simulink model "sim_tcyb_2024_pos_ctrl"  (R2020a)
settings: Solver=ode4  StartTime=0.0  StopTime=30.0  FixedStep=0.01  RelTol=1e-3
values from neighbouring files (symbols this model uses):
  alfa_theta = 20    [init_tcyb_2024_pos_ctrl.m]
  alfa_theta_obs = 100    [init_tcyb_2024_pos_ctrl.m]
  c1_diff_sigma_bar_v = diag([25; 30; 20])    [init_tcyb_2024_pos_ctrl.m]
  c1v = diag([5.8; 6.5; 6.5])    [init_tcyb_2024_pos_ctrl.m]
  c2_diff_sigma_bar_v = diag([50; 50; 10])    [init_tcyb_2024_pos_ctrl.m]
  c2v = diag([5.8; 6.5; 6.5])    [init_tcyb_2024_pos_ctrl.m]
  c3_diff_sigma_bar_v = diag([15; 15; 10])    [init_tcyb_2024_pos_ctrl.m]
  c3v = diag([4.8; 6.4; 6.0])    [init_tcyb_2024_pos_ctrl.m]
  c_psi_p = [0.05; 0.05; 0.05]    [init_tcyb_2024_pos_ctrl.m]
  delta_p_i_0 = zeros(3, NF)    [init_tcyb_2024_pos_ctrl.m]
  delta_v_i_0 = zeros(3, NF)    [init_tcyb_2024_pos_ctrl.m]
  dp_aa_t = 0.2 * ones(3, 5) + ( 1.0 - 0.2 ) * rand(3, 5)    [init_tcyb_2024_pos_ctrl.m]
  dp_ff_t = [ 0.4 * ones(1, 5) + ( 1.0 - 0.4 ) * rand(1, 5);                      0.4 * ones(1, 5) + ( 1.0 - 0.4 ) * rand(1, 5);                      0.2 * ones(1, 5) + ( 0.6 - 0.2 ) * rand(1, 5) ]    [init_tcyb_2024_pos_ctrl.m]
  dp_phi_t = ( - pi / 2 ) * ones(3, 5) + ( pi / 2 - ( - pi / 2 ) ) * rand(3, 5)    [init_tcyb_2024_pos_ctrl.m]
  etai_0 = zeros(3,5)    [init_tcyb_2024_pos_ctrl.m]
  kai_1_t = 0.02    [init_tcyb_2024_pos_ctrl.m]
  kai_3_t = 0.1    [init_tcyb_2024_pos_ctrl.m]
  ksii_0 = zeros(3,5)    [init_tcyb_2024_pos_ctrl.m]
  l1v = diag([20; 20; 20])    [init_tcyb_2024_pos_ctrl.m]
  l2v = diag([30; 30; 30])    [init_tcyb_2024_pos_ctrl.m]
  Lamd_diff_sigma_bar_v = 0.5    [init_tcyb_2024_pos_ctrl.m]
  mass_i = zeros(1,NF)    [init_tcyb_2024_pos_ctrl.m]
  Mii = diag([1;0;0;0;1])    [init_tcyb_2024_pos_ctrl.m]
  pos0 = zeros(3, 1)    [init_tcyb_2024_pos_ctrl.m]
  PZ0 = P0(3)    [init_tcyb_2024_pos_ctrl.m]
  PZ1 = 10    [init_tcyb_2024_pos_ctrl.m]
  Qci_init = repmat([1;0;0;0],1,NF)    [init_tcyb_2024_pos_ctrl.m]
  R0 = 4    [init_tcyb_2024_pos_ctrl.m]
  R1 = 8    [init_tcyb_2024_pos_ctrl.m]
  rho_p = [0.1; 0.1; 0.1]    [init_tcyb_2024_pos_ctrl.m]
  Rx2 = 10    [init_tcyb_2024_pos_ctrl.m]
  Ry2 = 6    [init_tcyb_2024_pos_ctrl.m]
  Rz2 = 4    [init_tcyb_2024_pos_ctrl.m]
  T0 = 0    [init_tcyb_2024_pos_ctrl.m]
  T1 = tseq1    (= 10)    [init_tcyb_2024_pos_ctrl.m]
  T12 = tseq1 + tseq12    (= 20)    [init_tcyb_2024_pos_ctrl.m]
  T2 = tseq1 + tseq12 + tseq2    (= 30)    [init_tcyb_2024_pos_ctrl.m]
  tau_p = 5    [init_tcyb_2024_pos_ctrl.m]
  theta0 = ( 2 / 5 ) * pi    (= 1.25663706144)    [init_tcyb_2024_pos_ctrl.m]
  vel0 = zeros(3, 1)    [init_tcyb_2024_pos_ctrl.m]
  Wij = [0,0,1,0,0;              0,0,1,1,0;              1,0,0,0,1;              0,1,1,0,0;              0,0,1,0,0]    [init_tcyb_2024_pos_ctrl.m]
  X1 = 8    [init_tcyb_2024_pos_ctrl.m]
  X2 = 2    [init_tcyb_2024_pos_ctrl.m]
  X3 = 3    [init_tcyb_2024_pos_ctrl.m]
  Y1 = 10    [init_tcyb_2024_pos_ctrl.m]
  Y2 = 2    [init_tcyb_2024_pos_ctrl.m]
  Y3 = 4    [init_tcyb_2024_pos_ctrl.m]
  Z1 = 4    [init_tcyb_2024_pos_ctrl.m]
  Z2 = -6    [init_tcyb_2024_pos_ctrl.m]
  Z3 = 2    [init_tcyb_2024_pos_ctrl.m]
  zeta_diff_sigma_bar_v = 0.08    [init_tcyb_2024_pos_ctrl.m]
undefined symbols (not defined in the file or in its folder): cal_frac_squ, p_alfav1, p_alfav2, p_gamma1_pos, p_gamma1_vel, p_gamma2_pos, p_gamma2_vel, q_alfav1, q_alfav2, q_gamma1_pos, q_gamma1_vel, q_gamma2_pos, q_gamma2_vel
(part 3 of 4)

== matlab function sim_tcyb_2024_pos_ctrl/cal theta_sigma_bar_v_tilt agent 3 ==
  data: alfa_theta input; sigma_bar_v_tilt_squ_1_3 input; theta_sigma_bar_v_tilt_1_3 output; sigma_bar_v_tilt_squ_2_3 input; sigma_bar_v_tilt_vec input; theta_sigma_bar_v_tilt_2_3 output
function [theta_sigma_bar_v_tilt_1_3, theta_sigma_bar_v_tilt_2_3] = fcn(alfa_theta, sigma_bar_v_tilt_squ_1_3, sigma_bar_v_tilt_squ_2_3, sigma_bar_v_tilt_vec)
%%%% 计算平滑递增函数
iiuav = 3;
theta_sigma_bar_v_tilt_1_3 = sigma_bar_v_tilt_squ_1_3(:) .* ( -1 + 2 ./ ( 1 + exp( -alfa_theta .* sigma_bar_v_tilt_vec(:,iiuav) ) ) );
theta_sigma_bar_v_tilt_2_3 = sigma_bar_v_tilt_squ_2_3(:) .* ( -1 + 2 ./ ( 1 + exp( -alfa_theta .* sigma_bar_v_tilt_vec(:,iiuav) ) ) );

== matlab function sim_tcyb_2024_pos_ctrl/choose ksi_est_err 25 ==
  data: x input; y output
function y = fcn(x)
iiuav = 3;
y = x(:,iiuav);

== matlab function sim_tcyb_2024_pos_ctrl/choose ksi_est_err 26 ==
  data: x input; y output
function y = fcn(x)
iiuav = 3;
y = x(:,iiuav);

== matlab function sim_tcyb_2024_pos_ctrl/trans to column24 ==
  data: x input; y output
function y = fcn(x)
y = x(:);

== matlab function sim_tcyb_2024_pos_ctrl/trans to column25 ==
  data: x input; y output
function y = fcn(x)
y = x(:);

== matlab function sim_tcyb_2024_pos_ctrl/cal abs 27 ==
  data: x input; y output
function y = fcn(x)
y = abs(x(:));

== matlab function sim_tcyb_2024_pos_ctrl/cal abs 28 ==
  data: x input; y output
function y = fcn(x)
y = abs(x(:));

== matlab function sim_tcyb_2024_pos_ctrl/cal theta_sigma_bar_v_tilt agent 4 ==
  data: alfa_theta input; sigma_bar_v_tilt_squ_1_4 input; theta_sigma_bar_v_tilt_1_4 output; sigma_bar_v_tilt_squ_2_4 input; sigma_bar_v_tilt_vec input; theta_sigma_bar_v_tilt_2_4 output
function [theta_sigma_bar_v_tilt_1_4, theta_sigma_bar_v_tilt_2_4] = fcn(alfa_theta, sigma_bar_v_tilt_squ_1_4, sigma_bar_v_tilt_squ_2_4, sigma_bar_v_tilt_vec)
%%%% 计算平滑递增函数
iiuav = 4;
theta_sigma_bar_v_tilt_1_4 = sigma_bar_v_tilt_squ_1_4(:) .* ( -1 + 2 ./ ( 1 + exp( -alfa_theta .* sigma_bar_v_tilt_vec(:,iiuav) ) ) );
theta_sigma_bar_v_tilt_2_4 = sigma_bar_v_tilt_squ_2_4(:) .* ( -1 + 2 ./ ( 1 + exp( -alfa_theta .* sigma_bar_v_tilt_vec(:,iiuav) ) ) );

== matlab function sim_tcyb_2024_pos_ctrl/choose ksi_est_err 27 ==
  data: x input; y output
function y = fcn(x)
iiuav = 4;
y = x(:,iiuav);

== matlab function sim_tcyb_2024_pos_ctrl/choose ksi_est_err 28 ==
  data: x input; y output
function y = fcn(x)
iiuav = 4;
y = x(:,iiuav);

== matlab function sim_tcyb_2024_pos_ctrl/cal lump formation error ==
  data: err_ksi_form_vec input; err_lump_vec output; err_eta_form_vec input
function err_lump_vec = fcn(err_ksi_form_vec, err_eta_form_vec)
%%%% 计算编队跟踪误差
err_lump_vec = zeros(3,5);
for iiuav = 1:5
    err_lump_vec(:,iiuav) = err_ksi_form_vec(:,iiuav) + err_eta_form_vec(:,iiuav);
end

== matlab function sim_tcyb_2024_pos_ctrl/trans to column26 ==
  data: x input; y output
function y = fcn(x)
y = x(:);

== matlab function sim_tcyb_2024_pos_ctrl/trans to column27 ==
  data: x input; y output
function y = fcn(x)
y = x(:);

== matlab function sim_tcyb_2024_pos_ctrl/cal abs 29 ==
  data: x input; y output
function y = fcn(x)
y = abs(x(:));

== matlab function sim_tcyb_2024_pos_ctrl/cal abs 30 ==
  data: x input; y output
function y = fcn(x)
y = abs(x(:));

== matlab function sim_tcyb_2024_pos_ctrl/cal theta_sigma_bar_v_tilt agent 5 ==
  data: alfa_theta input; sigma_bar_v_tilt_squ_1_5 input; theta_sigma_bar_v_tilt_1_5 output; sigma_bar_v_tilt_squ_2_5 input; sigma_bar_v_tilt_vec input; theta_sigma_bar_v_tilt_2_5 output
function [theta_sigma_bar_v_tilt_1_5, theta_sigma_bar_v_tilt_2_5] = fcn(alfa_theta, sigma_bar_v_tilt_squ_1_5, sigma_bar_v_tilt_squ_2_5, sigma_bar_v_tilt_vec)
%%%% 计算平滑递增函数
iiuav = 5;
theta_sigma_bar_v_tilt_1_5 = sigma_bar_v_tilt_squ_1_5(:) .* ( -1 + 2 ./ ( 1 + exp( -alfa_theta .* sigma_bar_v_tilt_vec(:,iiuav) ) ) );
theta_sigma_bar_v_tilt_2_5 = sigma_bar_v_tilt_squ_2_5(:) .* ( -1 + 2 ./ ( 1 + exp( -alfa_theta .* sigma_bar_v_tilt_vec(:,iiuav) ) ) );

== matlab function sim_tcyb_2024_pos_ctrl/choose ksi_est_err 29 ==
  data: x input; y output
function y = fcn(x)
iiuav = 5;
y = x(:,iiuav);

== matlab function sim_tcyb_2024_pos_ctrl/choose ksi_est_err 30 ==
  data: x input; y output
function y = fcn(x)
iiuav = 5;
y = x(:,iiuav);

== matlab function sim_tcyb_2024_pos_ctrl/trans to column28 ==
  data: x input; y output
function y = fcn(x)
y = x(:);

== matlab function sim_tcyb_2024_pos_ctrl/trans to column29 ==
  data: x input; y output
function y = fcn(x)
y = x(:);

== matlab function sim_tcyb_2024_pos_ctrl/combine theta_sigma_bar_v_tilt ==
  data: theta_sigma_bar_v_tilt_1_1 input; theta_sigma_bar_v_tilt_1_2 input; theta_sigma_bar_v_tilt_1_3 input; theta_sigma_bar_v_tilt_1_4 input; theta_sigma_bar_v_tilt_1_5 input; theta_sigma_bar_v_tilt_1_vec output; theta_sigma_bar_v_tilt_2_1 input; theta_sigma_bar_v_tilt_2_vec output; theta_sigma_bar_v_tilt_2_2 input; theta_sigma_bar_v_tilt_2_3 input; theta_sigma_bar_v_tilt_2_4 input; theta_sigma_bar_v_tilt_2_5 input
function [theta_sigma_bar_v_tilt_1_vec, theta_sigma_bar_v_tilt_2_vec]  = fcn(theta_sigma_bar_v_tilt_1_1, theta_sigma_bar_v_tilt_1_2, theta_sigma_bar_v_tilt_1_3, theta_sigma_bar_v_tilt_1_4, theta_sigma_bar_v_tilt_1_5, ...
                                                                                                                                            theta_sigma_bar_v_tilt_2_1, theta_sigma_bar_v_tilt_2_2, theta_sigma_bar_v_tilt_2_3, theta_sigma_bar_v_tilt_2_4, theta_sigma_bar_v_tilt_2_5)
%%%% 合并领导者位置观测器输出结果
theta_sigma_bar_v_tilt_1_vec = [theta_sigma_bar_v_tilt_1_1(:), theta_sigma_bar_v_tilt_1_2(:), theta_sigma_bar_v_tilt_1_3(:), theta_sigma_bar_v_tilt_1_4(:), theta_sigma_bar_v_tilt_1_5(:)];
theta_sigma_bar_v_tilt_2_vec = [theta_sigma_bar_v_tilt_2_1(:), theta_sigma_bar_v_tilt_2_2(:), theta_sigma_bar_v_tilt_2_3(:), theta_sigma_bar_v_tilt_2_4(:), theta_sigma_bar_v_tilt_2_5(:)];

== matlab function sim_tcyb_2024_pos_ctrl/eps_p_hat adaptive law agent 1 ==
  data: rho_p input; d_eps_p_hat_1 output; err_lump_vec input
function d_eps_p_hat_1 = fcn(rho_p, err_lump_vec)
%%%% 计算自适应律
iiuav = 1;
d_eps_p_hat_1 = ( rho_p(:) .* err_lump_vec(:,iiuav) )' * err_lump_vec(:,iiuav);

== matlab function sim_tcyb_2024_pos_ctrl/cal sigma_bar_v_hat agent 1 ==
  data: c1v input; c2v input; theta_sigma_bar_v_tilt_1_vec input; d_sigma_bar_v_hat_1 output; theta_sigma_bar_v_tilt_2_vec input; d_sigma_bar_v_vec input
function d_sigma_bar_v_hat_1 = fcn(c1v, c2v, theta_sigma_bar_v_tilt_1_vec, theta_sigma_bar_v_tilt_2_vec, d_sigma_bar_v_vec)
%%%% 计算扰动观测器中虚拟速度控制量观测值sigma_v_hat的微分方程
iiuav = 1;
d_sigma_bar_v_hat_1 = d_sigma_bar_v_vec(:,iiuav) + ...
                                            c1v * theta_sigma_bar_v_tilt_1_vec(:,iiuav) + ...
                                            c2v * theta_sigma_bar_v_tilt_2_vec(:,iiuav);

== matlab function sim_tcyb_2024_pos_ctrl/cal sigma_bar_v_hat agent 2 ==
  data: c1v input; c2v input; theta_sigma_bar_v_tilt_1_vec input; d_sigma_bar_v_hat_2 output; theta_sigma_bar_v_tilt_2_vec input; d_sigma_bar_v_vec input
function d_sigma_bar_v_hat_2 = fcn(c1v, c2v, theta_sigma_bar_v_tilt_1_vec, theta_sigma_bar_v_tilt_2_vec, d_sigma_bar_v_vec)
%%%% 计算扰动观测器中虚拟速度控制量观测值sigma_v_hat的微分方程
iiuav = 2;
d_sigma_bar_v_hat_2 = d_sigma_bar_v_vec(:,iiuav) + ...
                                            c1v * theta_sigma_bar_v_tilt_1_vec(:,iiuav) + ...
                                            c2v * theta_sigma_bar_v_tilt_2_vec(:,iiuav);

== matlab function sim_tcyb_2024_pos_ctrl/cal sigma_bar_v_hat agent 3 ==
  data: c1v input; c2v input; theta_sigma_bar_v_tilt_1_vec input; d_sigma_bar_v_hat_3 output; theta_sigma_bar_v_tilt_2_vec input; d_sigma_bar_v_vec input
function d_sigma_bar_v_hat_3 = fcn(c1v, c2v, theta_sigma_bar_v_tilt_1_vec, theta_sigma_bar_v_tilt_2_vec, d_sigma_bar_v_vec)
%%%% 计算扰动观测器中虚拟速度控制量观测值sigma_v_hat的微分方程
iiuav = 3;
d_sigma_bar_v_hat_3 = d_sigma_bar_v_vec(:,iiuav) + ...
                                            c1v * theta_sigma_bar_v_tilt_1_vec(:,iiuav) + ...
                                            c2v * theta_sigma_bar_v_tilt_2_vec(:,iiuav);

== matlab function sim_tcyb_2024_pos_ctrl/cal sigma_bar_v_hat agent 4 ==
  data: c1v input; c2v input; theta_sigma_bar_v_tilt_1_vec input; d_sigma_bar_v_hat_4 output; theta_sigma_bar_v_tilt_2_vec input; d_sigma_bar_v_vec input
function d_sigma_bar_v_hat_4 = fcn(c1v, c2v, theta_sigma_bar_v_tilt_1_vec, theta_sigma_bar_v_tilt_2_vec, d_sigma_bar_v_vec)
%%%% 计算扰动观测器中虚拟速度控制量观测值sigma_v_hat的微分方程
iiuav = 4;
d_sigma_bar_v_hat_4 = d_sigma_bar_v_vec(:,iiuav) + ...
                                            c1v * theta_sigma_bar_v_tilt_1_vec(:,iiuav) + ...
                                            c2v * theta_sigma_bar_v_tilt_2_vec(:,iiuav);

== matlab function sim_tcyb_2024_pos_ctrl/cal sigma_bar_v_hat agent 5 ==
  data: c1v input; c2v input; theta_sigma_bar_v_tilt_1_vec input; d_sigma_bar_v_hat_5 output; theta_sigma_bar_v_tilt_2_vec input; d_sigma_bar_v_vec input
function d_sigma_bar_v_hat_5 = fcn(c1v, c2v, theta_sigma_bar_v_tilt_1_vec, theta_sigma_bar_v_tilt_2_vec, d_sigma_bar_v_vec)
%%%% 计算扰动观测器中虚拟速度控制量观测值sigma_v_hat的微分方程
iiuav = 5;
d_sigma_bar_v_hat_5 = d_sigma_bar_v_vec(:,iiuav) + ...
                                            c1v * theta_sigma_bar_v_tilt_1_vec(:,iiuav) + ...
                                            c2v * theta_sigma_bar_v_tilt_2_vec(:,iiuav);

== matlab function sim_tcyb_2024_pos_ctrl/cal combine sigma_bar_v_tilt ==
  data: sigma_bar_v_vec input; sigma_bar_v_hat_vec input; sigma_bar_v_tilt_vec output
function sigma_bar_v_tilt_vec = fcn(sigma_bar_v_vec, sigma_bar_v_hat_vec)
%%%% 计算虚拟速度观测误差sigma_bar_v_tilt
sigma_bar_v_tilt_vec = zeros(3,5);
for iiuav = 1:5
    sigma_bar_v_tilt_vec(:,iiuav) = sigma_bar_v_vec(:,iiuav) - sigma_bar_v_hat_vec(:,iiuav);
end

== matlab function sim_tcyb_2024_pos_ctrl/combine sigma_bar_v_hat ==
  data: sigma_bar_v_hat_1 input; sigma_bar_v_hat_2 input; sigma_bar_v_hat_3 input; sigma_bar_v_hat_4 input; sigma_bar_v_hat_5 input; sigma_bar_v_hat_vec output
function sigma_bar_v_hat_vec  = fcn(sigma_bar_v_hat_1, sigma_bar_v_hat_2, sigma_bar_v_hat_3, sigma_bar_v_hat_4, sigma_bar_v_hat_5)
%%%% 合并虚拟速度控制量观测值sigma_bar_v_hat
sigma_bar_v_hat_vec = [sigma_bar_v_hat_1(:), sigma_bar_v_hat_2(:), sigma_bar_v_hat_3(:), sigma_bar_v_hat_4(:), sigma_bar_v_hat_5(:)];

== matlab function sim_tcyb_2024_pos_ctrl/cal formation tracking position errors ==
  data: wi0 input; err_ksi_form_vec output; wij input; err_ksi_vec input
function err_ksi_form_vec = fcn(wi0, wij, err_ksi_vec)
%%%% 计算编队跟踪误差
err_ksi_form_vec = zeros(3,5);
for iiuav = 1:5
    err_ksi_form_vec(:,iiuav) = wi0(iiuav, iiuav) * err_ksi_vec(:,iiuav);
    for jjuav = 1:5
        err_ksi_form_vec(:,iiuav) = err_ksi_form_vec(:,iiuav) ...
                                                        + wij(iiuav, jjuav) * (err_ksi_vec(:,iiuav) - err_ksi_vec(:,jjuav));
    end
end

== matlab function sim_tcyb_2024_pos_ctrl/cal dp_hat agent 1 ==
  data: c3v input; d_sigma_bar_v_vec input; sigma_bar_v_hat_vec input; dp_hat_1 output
function dp_hat_1 = fcn(c3v, d_sigma_bar_v_vec, sigma_bar_v_hat_vec)
%%%% 计算扰动观测值dp_hat
iiuav = 1;
dp_hat_1 = d_sigma_bar_v_vec(:,iiuav) + c3v * sigma_bar_v_hat_vec(:,iiuav);

== matlab function sim_tcyb_2024_pos_ctrl/cal dp_hat agent 2 ==
  data: c3v input; d_sigma_bar_v_vec input; sigma_bar_v_hat_vec input; dp_hat_2 output
function dp_hat_2 = fcn(c3v, d_sigma_bar_v_vec, sigma_bar_v_hat_vec)
%%%% 计算扰动观测值dp_hat
iiuav = 2;
dp_hat_2 = d_sigma_bar_v_vec(:,iiuav) + c3v * sigma_bar_v_hat_vec(:,iiuav);

== matlab function sim_tcyb_2024_pos_ctrl/cal dp_hat agent 3 ==
  data: c3v input; d_sigma_bar_v_vec input; sigma_bar_v_hat_vec input; dp_hat_3 output
function dp_hat_3 = fcn(c3v, d_sigma_bar_v_vec, sigma_bar_v_hat_vec)
%%%% 计算扰动观测值dp_hat
iiuav = 3;
dp_hat_3 = d_sigma_bar_v_vec(:,iiuav) + c3v * sigma_bar_v_hat_vec(:,iiuav);

== matlab function sim_tcyb_2024_pos_ctrl/cal dp_hat agent 4 ==
  data: c3v input; d_sigma_bar_v_vec input; sigma_bar_v_hat_vec input; dp_hat_4 output
function dp_hat_4 = fcn(c3v, d_sigma_bar_v_vec, sigma_bar_v_hat_vec)
%%%% 计算扰动观测值dp_hat
iiuav = 4;
dp_hat_4 = d_sigma_bar_v_vec(:,iiuav) + c3v * sigma_bar_v_hat_vec(:,iiuav);

== matlab function sim_tcyb_2024_pos_ctrl/cal dp_hat agent 5 ==
  data: c3v input; d_sigma_bar_v_vec input; sigma_bar_v_hat_vec input; dp_hat_5 output
function dp_hat_5 = fcn(c3v, d_sigma_bar_v_vec, sigma_bar_v_hat_vec)
%%%% 计算扰动观测值dp_hat
iiuav = 5;
dp_hat_5 = d_sigma_bar_v_vec(:,iiuav) + c3v * sigma_bar_v_hat_vec(:,iiuav);

== matlab function sim_tcyb_2024_pos_ctrl/combine dp_hat ==
  data: dp_hat_1 input; dp_hat_2 input; dp_hat_3 input; dp_hat_4 input; dp_hat_5 input; dp_hat_vec output
function dp_hat_vec  = fcn(dp_hat_1, dp_hat_2, dp_hat_3, dp_hat_4, dp_hat_5)
%%%% 合并扰动观测值dp_hat
dp_hat_vec = [dp_hat_1(:), dp_hat_2(:), dp_hat_3(:), dp_hat_4(:), dp_hat_5(:)];

== matlab function sim_tcyb_2024_pos_ctrl/cal ui agent 1 ==
  data: c_psi_p input; d_delta_eta_vec input; ui_1 output; err_Gi_form_vec input; eps_p_hat_vec input; err_lump_vec input; dp_hat_vec input
function ui_1 = fcn(c_psi_p, d_delta_eta_vec, err_Gi_form_vec, eps_p_hat_vec, err_lump_vec, dp_hat_vec)
%%%% 计算控制输入ui
iiuav = 1;
g0 = 9.80663;
e3 = [0;0;1];
ui_1 = g0 * e3 + d_delta_eta_vec(:,iiuav) - c_psi_p(:) .* err_Gi_form_vec(:,iiuav) ...
            - eps_p_hat_vec(iiuav) * err_lump_vec(:,iiuav) - dp_hat_vec(:,iiuav);

== matlab function sim_tcyb_2024_pos_ctrl/combine ui ==
  data: ui_1 input; ui_2 input; ui_3 input; ui_4 input; ui_5 input; ui_vec output
function ui_vec  = fcn(ui_1, ui_2, ui_3, ui_4, ui_5)
%%%% 合并控制输入ui
ui_vec = [ui_1(:), ui_2(:), ui_3(:), ui_4(:), ui_5(:)];

== matlab function sim_tcyb_2024_pos_ctrl/cal disturbance observation error dp_tilt ==
  data: dp_vec input; dp_tilt_vec output; dp_hat_vec input
function dp_tilt_vec = fcn(dp_vec, dp_hat_vec)
%%%% 计算扰动观测器估计误差dp_tilt
dp_tilt_vec = zeros(3,5);
for iiuav = 1:5
    dp_tilt_vec(:,iiuav) = dp_vec(:,iiuav) - dp_hat_vec(:,iiuav);
end

== matlab function sim_tcyb_2024_pos_ctrl/cal abs 41 ==
  data: x input; y output
function y = fcn(x)
y = abs(x(:));

== matlab function sim_tcyb_2024_pos_ctrl/eps_p_hat adaptive law agent 2 ==
  data: rho_p input; d_eps_p_hat_2 output; err_lump_vec input
function d_eps_p_hat_2 = fcn(rho_p, err_lump_vec)
%%%% 计算自适应律
iiuav = 2;
d_eps_p_hat_2 = ( rho_p(:) .* err_lump_vec(:,iiuav) )' * err_lump_vec(:,iiuav);

== matlab function sim_tcyb_2024_pos_ctrl/cal abs 42 ==
  data: x input; y output
function y = fcn(x)
y = abs(x(:));

== matlab function sim_tcyb_2024_pos_ctrl/cal abs 43 ==
  data: x input; y output
function y = fcn(x)
y = abs(x(:));

== matlab function sim_tcyb_2024_pos_ctrl/cal abs 44 ==
  data: x input; y output
function y = fcn(x)
y = abs(x(:));

== matlab function sim_tcyb_2024_pos_ctrl/cal abs 45 ==
  data: x input; y output
function y = fcn(x)
y = abs(x(:));

== matlab function sim_tcyb_2024_pos_ctrl/cal abs 46 ==
  data: x input; y output
function y = fcn(x)
y = abs(x(:));

== matlab function sim_tcyb_2024_pos_ctrl/cal abs 47 ==
  data: x input; y output
function y = fcn(x)
y = abs(x(:));

== matlab function sim_tcyb_2024_pos_ctrl/cal abs 48 ==
  data: x input; y output
function y = fcn(x)
y = abs(x(:));

== matlab function sim_tcyb_2024_pos_ctrl/cal abs 49 ==
  data: x input; y output
function y = fcn(x)
y = abs(x(:));

== matlab function sim_tcyb_2024_pos_ctrl/cal abs 50 ==
  data: x input; y output
function y = fcn(x)
y = abs(x(:));

== matlab function sim_tcyb_2024_pos_ctrl/cal abs 51 ==
  data: x input; y output
function y = fcn(x)
y = abs(x(:));

== matlab function sim_tcyb_2024_pos_ctrl/cal abs 52 ==
  data: x input; y output
function y = fcn(x)
y = abs(x(:));

== matlab function sim_tcyb_2024_pos_ctrl/eps_p_hat adaptive law agent 3 ==
  data: rho_p input; d_eps_p_hat_3 output; err_lump_vec input
function d_eps_p_hat_3 = fcn(rho_p, err_lump_vec)
%%%% 计算自适应律
iiuav = 3;
d_eps_p_hat_3 = ( rho_p(:) .* err_lump_vec(:,iiuav) )' * err_lump_vec(:,iiuav);

== matlab function sim_tcyb_2024_pos_ctrl/cal abs 53 ==
  data: x input; y output
function y = fcn(x)
y = abs(x(:));

== matlab function sim_tcyb_2024_pos_ctrl/cal abs 54 ==
  data: x input; y output
function y = fcn(x)
y = abs(x(:));

== matlab function sim_tcyb_2024_pos_ctrl/cal abs 55 ==
  data: x input; y output
function y = fcn(x)
y = abs(x(:));

== matlab function sim_tcyb_2024_pos_ctrl/cal abs 56 ==
  data: x input; y output
function y = fcn(x)
y = abs(x(:));

== matlab function sim_tcyb_2024_pos_ctrl/cal abs 57 ==
  data: x input; y output
function y = fcn(x)
y = abs(x(:));

== matlab function sim_tcyb_2024_pos_ctrl/cal abs 58 ==
  data: x input; y output
function y = fcn(x)
y = abs(x(:));

== matlab function sim_tcyb_2024_pos_ctrl/cal abs 59 ==
  data: x input; y output
function y = fcn(x)
y = abs(x(:));

== matlab function sim_tcyb_2024_pos_ctrl/cal abs 60 ==
  data: x input; y output
function y = fcn(x)
y = abs(x(:));

== matlab function sim_tcyb_2024_pos_ctrl/cal lumped observation error agent 1 ==
  data: wij input; w0 input; ksi_d_est_vec input; ksi0 input; delta_ksi_vec input; eta_d_est_vec input; ksi_est_err_tilt_1 output; eta0 input; delta_eta_vec input; eta_est_err_tilt_1 output
function [ksi_est_err_tilt_1, eta_est_err_tilt_1]  = fcn(wij, w0, ksi_d_est_vec, ksi0, delta_ksi_vec, eta_d_est_vec, eta0, delta_eta_vec)
%%%% 计算跟随者期望速度分布式观测器误差
iiuav = 1;
ksi_est_err_tilt_1 = w0(iiuav, iiuav) * (ksi_d_est_vec(:,iiuav) - ksi0(:) - delta_ksi_vec(:,iiuav));
eta_est_err_tilt_1 = w0(iiuav, iiuav) * (eta_d_est_vec(:,iiuav) - eta0(:) - delta_eta_vec(:,iiuav));
for jjuav = 1:5
    ksi_est_err_tilt_1 = ksi_est_err_tilt_1 + ...
                                        wij(iiuav, jjuav) * ((ksi_d_est_vec(:,iiuav) - delta_ksi_vec(:,iiuav)) - (ksi_d_est_vec(:,jjuav) - delta_ksi_vec(:,jjuav)));
    eta_est_err_tilt_1 = eta_est_err_tilt_1 + ...
                                        wij(iiuav, jjuav) * ((eta_d_est_vec(:,iiuav) - delta_eta_vec(:,iiuav)) - (eta_d_est_vec(:,jjuav) - delta_eta_vec(:,jjuav)));
end

== matlab function sim_tcyb_2024_pos_ctrl/cal lumped observation error agent 2 ==
  data: wij input; w0 input; ksi_d_est_vec input; ksi0 input; delta_ksi_vec input; eta_d_est_vec input; ksi_est_err_tilt_2 output; eta0 input; delta_eta_vec input; eta_est_err_tilt_2 output
function [ksi_est_err_tilt_2, eta_est_err_tilt_2]  = fcn(wij, w0, ksi_d_est_vec, ksi0, delta_ksi_vec, eta_d_est_vec, eta0, delta_eta_vec)
%%%% 计算跟随者期望速度分布式观测器误差
iiuav = 2;
ksi_est_err_tilt_2 = w0(iiuav, iiuav) * (ksi_d_est_vec(:,iiuav) - ksi0(:) - delta_ksi_vec(:,iiuav));
eta_est_err_tilt_2 = w0(iiuav, iiuav) * (eta_d_est_vec(:,iiuav) - eta0(:) - delta_eta_vec(:,iiuav));
for jjuav = 1:5
    ksi_est_err_tilt_2 = ksi_est_err_tilt_2 + ...
                                        wij(iiuav, jjuav) * ((ksi_d_est_vec(:,iiuav) - delta_ksi_vec(:,iiuav)) - (ksi_d_est_vec(:,jjuav) - delta_ksi_vec(:,jjuav)));
    eta_est_err_tilt_2 = eta_est_err_tilt_2 + ...
                                        wij(iiuav, jjuav) * ((eta_d_est_vec(:,iiuav) - delta_eta_vec(:,iiuav)) - (eta_d_est_vec(:,jjuav) - delta_eta_vec(:,jjuav)));
end

== matlab function sim_tcyb_2024_pos_ctrl/eps_p_hat adaptive law agent 4 ==
  data: rho_p input; d_eps_p_hat_4 output; err_lump_vec input
function d_eps_p_hat_4 = fcn(rho_p, err_lump_vec)
%%%% 计算自适应律
iiuav = 4;
d_eps_p_hat_4 = ( rho_p(:) .* err_lump_vec(:,iiuav) )' * err_lump_vec(:,iiuav);

== matlab function sim_tcyb_2024_pos_ctrl/cal lumped observation error agent 3 ==
  data: wij input; w0 input; ksi_d_est_vec input; ksi0 input; delta_ksi_vec input; eta_d_est_vec input; ksi_est_err_tilt_3 output; eta0 input; delta_eta_vec input; eta_est_err_tilt_3 output
function [ksi_est_err_tilt_3, eta_est_err_tilt_3]  = fcn(wij, w0, ksi_d_est_vec, ksi0, delta_ksi_vec, eta_d_est_vec, eta0, delta_eta_vec)
%%%% 计算跟随者期望速度分布式观测器误差
iiuav = 3;
ksi_est_err_tilt_3 = w0(iiuav, iiuav) * (ksi_d_est_vec(:,iiuav) - ksi0(:) - delta_ksi_vec(:,iiuav));
eta_est_err_tilt_3 = w0(iiuav, iiuav) * (eta_d_est_vec(:,iiuav) - eta0(:) - delta_eta_vec(:,iiuav));
for jjuav = 1:5
    ksi_est_err_tilt_3 = ksi_est_err_tilt_3 + ...
                                        wij(iiuav, jjuav) * ((ksi_d_est_vec(:,iiuav) - delta_ksi_vec(:,iiuav)) - (ksi_d_est_vec(:,jjuav) - delta_ksi_vec(:,jjuav)));
    eta_est_err_tilt_3 = eta_est_err_tilt_3 + ...
                                        wij(iiuav, jjuav) * ((eta_d_est_vec(:,iiuav) - delta_eta_vec(:,iiuav)) - (eta_d_est_vec(:,jjuav) - delta_eta_vec(:,jjuav)));
end

== matlab function sim_tcyb_2024_pos_ctrl/cal lumped observation error agent 4 ==
  data: wij input; w0 input; ksi_d_est_vec input; ksi0 input; delta_ksi_vec input; eta_d_est_vec input; ksi_est_err_tilt_4 output; eta0 input; delta_eta_vec input; eta_est_err_tilt_4 output
function [ksi_est_err_tilt_4, eta_est_err_tilt_4]  = fcn(wij, w0, ksi_d_est_vec, ksi0, delta_ksi_vec, eta_d_est_vec, eta0, delta_eta_vec)
%%%% 计算跟随者期望速度分布式观测器误差
iiuav = 4;
ksi_est_err_tilt_4 = w0(iiuav, iiuav) * (ksi_d_est_vec(:,iiuav) - ksi0(:) - delta_ksi_vec(:,iiuav));
eta_est_err_tilt_4 = w0(iiuav, iiuav) * (eta_d_est_vec(:,iiuav) - eta0(:) - delta_eta_vec(:,iiuav));
for jjuav = 1:5
    ksi_est_err_tilt_4 = ksi_est_err_tilt_4 + ...
                                        wij(iiuav, jjuav) * ((ksi_d_est_vec(:,iiuav) - delta_ksi_vec(:,iiuav)) - (ksi_d_est_vec(:,jjuav) - delta_ksi_vec(:,jjuav)));
    eta_est_err_tilt_4 = eta_est_err_tilt_4 + ...
                                        wij(iiuav, jjuav) * ((eta_d_est_vec(:,iiuav) - delta_eta_vec(:,iiuav)) - (eta_d_est_vec(:,jjuav) - delta_eta_vec(:,jjuav)));
end

== matlab function sim_tcyb_2024_pos_ctrl/cal lumped observation error agent 5 ==
  data: wij input; w0 input; ksi_d_est_vec input; ksi0 input; delta_ksi_vec input; eta_d_est_vec input; ksi_est_err_tilt_5 output; eta0 input; delta_eta_vec input; eta_est_err_tilt_5 output
function [ksi_est_err_tilt_5, eta_est_err_tilt_5]  = fcn(wij, w0, ksi_d_est_vec, ksi0, delta_ksi_vec, eta_d_est_vec, eta0, delta_eta_vec)
%%%% 计算跟随者期望速度分布式观测器误差
iiuav = 5;
ksi_est_err_tilt_5 = w0(iiuav, iiuav) * (ksi_d_est_vec(:,iiuav) - ksi0(:) - delta_ksi_vec(:,iiuav));
eta_est_err_tilt_5 = w0(iiuav, iiuav) * (eta_d_est_vec(:,iiuav) - eta0(:) - delta_eta_vec(:,iiuav));
for jjuav = 1:5
    ksi_est_err_tilt_5 = ksi_est_err_tilt_5 + ...
                                        wij(iiuav, jjuav) * ((ksi_d_est_vec(:,iiuav) - delta_ksi_vec(:,iiuav)) - (ksi_d_est_vec(:,jjuav) - delta_ksi_vec(:,jjuav)));
    eta_est_err_tilt_5 = eta_est_err_tilt_5 + ...
                                        wij(iiuav, jjuav) * ((eta_d_est_vec(:,iiuav) - delta_eta_vec(:,iiuav)) - (eta_d_est_vec(:,jjuav) - delta_eta_vec(:,jjuav)));
end

== matlab function sim_tcyb_2024_pos_ctrl/cal position estimate error ==
  data: ksi_d_est_vec input; ksi_est_err output; ksi0 input; delta_ksi_vec input
function ksi_est_err  = fcn(ksi_d_est_vec, ksi0, delta_ksi_vec)
%%%% 计算跟随者期望位置分布式观测器误差
ksi_est_err = ksi_d_est_vec - repmat(ksi0, 1, 5) - delta_ksi_vec;

== matlab function sim_tcyb_2024_pos_ctrl/cal theta_eta_est_err_tilt agent 1 ==
  data: alfa_theta input; eta_est_err_squ_1_node_1 input; theta_eta_est_err_tilt_1_1 output; eta_est_err_squ_2_node_1 input; eta_est_err_tilt_vec input; theta_eta_est_err_tilt_2_1 output
function [theta_eta_est_err_tilt_1_1, theta_eta_est_err_tilt_2_1] = fcn(alfa_theta, eta_est_err_squ_1_node_1, eta_est_err_squ_2_node_1, eta_est_err_tilt_vec)
%%%% 计算平滑递增函数
iiuav = 1;
theta_eta_est_err_tilt_1_1 = eta_est_err_squ_1_node_1(:) .* ( -1 + 2 ./ ( 1 + exp( -alfa_theta .* eta_est_err_tilt_vec(:,iiuav) ) ) );
theta_eta_est_err_tilt_2_1 = eta_est_err_squ_2_node_1(:) .* ( -1 + 2 ./ ( 1 + exp( -alfa_theta .* eta_est_err_tilt_vec(:,iiuav) ) ) );

== matlab function sim_tcyb_2024_pos_ctrl/cal theta_eta_est_err_tilt agent 2 ==
  data: alfa_theta input; eta_est_err_squ_1_node_2 input; theta_eta_est_err_tilt_1_2 output; eta_est_err_squ_2_node_2 input; eta_est_err_tilt_vec input; theta_eta_est_err_tilt_2_2 output
function [theta_eta_est_err_tilt_1_2, theta_eta_est_err_tilt_2_2] = fcn(alfa_theta, eta_est_err_squ_1_node_2, eta_est_err_squ_2_node_2, eta_est_err_tilt_vec)
%%%% 计算平滑递增函数
iiuav = 2;
theta_eta_est_err_tilt_1_2 = eta_est_err_squ_1_node_2(:) .* ( -1 + 2 ./ ( 1 + exp( -alfa_theta .* eta_est_err_tilt_vec(:,iiuav) ) ) );
theta_eta_est_err_tilt_2_2 = eta_est_err_squ_2_node_2(:) .* ( -1 + 2 ./ ( 1 + exp( -alfa_theta .* eta_est_err_tilt_vec(:,iiuav) ) ) );

== matlab function sim_tcyb_2024_pos_ctrl/eps_p_hat adaptive law agent 5 ==
  data: rho_p input; d_eps_p_hat_5 output; err_lump_vec input
function d_eps_p_hat_5 = fcn(rho_p, err_lump_vec)
%%%% 计算自适应律
iiuav = 5;
d_eps_p_hat_5 = ( rho_p(:) .* err_lump_vec(:,iiuav) )' * err_lump_vec(:,iiuav);

== matlab function sim_tcyb_2024_pos_ctrl/cal theta_eta_est_err_tilt agent 3 ==
  data: alfa_theta input; eta_est_err_squ_1_node_3 input; theta_eta_est_err_tilt_1_3 output; eta_est_err_squ_2_node_3 input; eta_est_err_tilt_vec input; theta_eta_est_err_tilt_2_3 output
function [theta_eta_est_err_tilt_1_3, theta_eta_est_err_tilt_2_3] = fcn(alfa_theta, eta_est_err_squ_1_node_3, eta_est_err_squ_2_node_3, eta_est_err_tilt_vec)
%%%% 计算平滑递增函数
iiuav = 3;
theta_eta_est_err_tilt_1_3 = eta_est_err_squ_1_node_3(:) .* ( -1 + 2 ./ ( 1 + exp( -alfa_theta .* eta_est_err_tilt_vec(:,iiuav) ) ) );
theta_eta_est_err_tilt_2_3 = eta_est_err_squ_2_node_3(:) .* ( -1 + 2 ./ ( 1 + exp( -alfa_theta .* eta_est_err_tilt_vec(:,iiuav) ) ) );

== matlab function sim_tcyb_2024_pos_ctrl/cal theta_eta_est_err_tilt agent 4 ==
  data: alfa_theta input; eta_est_err_squ_1_node_4 input; theta_eta_est_err_tilt_1_4 output; eta_est_err_squ_2_node_4 input; eta_est_err_tilt_vec input; theta_eta_est_err_tilt_2_4 output
function [theta_eta_est_err_tilt_1_4, theta_eta_est_err_tilt_2_4] = fcn(alfa_theta, eta_est_err_squ_1_node_4, eta_est_err_squ_2_node_4, eta_est_err_tilt_vec)
%%%% 计算平滑递增函数
iiuav = 4;
theta_eta_est_err_tilt_1_4 = eta_est_err_squ_1_node_4(:) .* ( -1 + 2 ./ ( 1 + exp( -alfa_theta .* eta_est_err_tilt_vec(:,iiuav) ) ) );
theta_eta_est_err_tilt_2_4 = eta_est_err_squ_2_node_4(:) .* ( -1 + 2 ./ ( 1 + exp( -alfa_theta .* eta_est_err_tilt_vec(:,iiuav) ) ) );

== matlab function sim_tcyb_2024_pos_ctrl/cal theta_eta_est_err_tilt agent 5 ==
  data: alfa_theta input; eta_est_err_squ_1_node_5 input; theta_eta_est_err_tilt_1_5 output; eta_est_err_squ_2_node_5 input; eta_est_err_tilt_vec input; theta_eta_est_err_tilt_2_5 output
function [theta_eta_est_err_tilt_1_5, theta_eta_est_err_tilt_2_5] = fcn(alfa_theta, eta_est_err_squ_1_node_5, eta_est_err_squ_2_node_5, eta_est_err_tilt_vec)
%%%% 计算平滑递增函数
iiuav = 5;
theta_eta_est_err_tilt_1_5 = eta_est_err_squ_1_node_5(:) .* ( -1 + 2 ./ ( 1 + exp( -alfa_theta .* eta_est_err_tilt_vec(:,iiuav) ) ) );
theta_eta_est_err_tilt_2_5 = eta_est_err_squ_2_node_5(:) .* ( -1 + 2 ./ ( 1 + exp( -alfa_theta .* eta_est_err_tilt_vec(:,iiuav) ) ) );

== matlab function sim_tcyb_2024_pos_ctrl/cal theta_ksi_est_err_tilt agent 1 ==
  data: alfa_theta input; ksi_est_err_squ_1_node_1 input; theta_ksi_est_err_tilt_1_1 output; ksi_est_err_squ_2_node_1 input; ksi_est_err_tilt_vec input; theta_ksi_est_err_tilt_2_1 output
function [theta_ksi_est_err_tilt_1_1, theta_ksi_est_err_tilt_2_1] = fcn(alfa_theta, ksi_est_err_squ_1_node_1, ksi_est_err_squ_2_node_1, ksi_est_err_tilt_vec)
%%%% 计算平滑递增函数
iiuav = 1;
theta_ksi_est_err_tilt_1_1 = ksi_est_err_squ_1_node_1(:) .* ( -1 + 2 ./ ( 1 + exp( -alfa_theta .* ksi_est_err_tilt_vec(:,iiuav) ) ) );
theta_ksi_est_err_tilt_2_1 = ksi_est_err_squ_2_node_1(:) .* ( -1 + 2 ./ ( 1 + exp( -alfa_theta .* ksi_est_err_tilt_vec(:,iiuav) ) ) );

== matlab function sim_tcyb_2024_pos_ctrl/cal theta_ksi_est_err_tilt agent 2 ==
  data: alfa_theta input; ksi_est_err_squ_1_node_2 input; theta_ksi_est_err_tilt_1_2 output; ksi_est_err_squ_2_node_2 input; ksi_est_err_tilt_vec input; theta_ksi_est_err_tilt_2_2 output
function [theta_ksi_est_err_tilt_1_2, theta_ksi_est_err_tilt_2_2] = fcn(alfa_theta, ksi_est_err_squ_1_node_2, ksi_est_err_squ_2_node_2, ksi_est_err_tilt_vec)
%%%% 计算平滑递增函数
iiuav = 2;
theta_ksi_est_err_tilt_1_2 = ksi_est_err_squ_1_node_2(:) .* ( -1 + 2 ./ ( 1 + exp( -alfa_theta .* ksi_est_err_tilt_vec(:,iiuav) ) ) );
theta_ksi_est_err_tilt_2_2 = ksi_est_err_squ_2_node_2(:) .* ( -1 + 2 ./ ( 1 + exp( -alfa_theta .* ksi_est_err_tilt_vec(:,iiuav) ) ) );

== matlab function sim_tcyb_2024_pos_ctrl/cal theta_ksi_est_err_tilt agent 3 ==
  data: alfa_theta input; ksi_est_err_squ_1_node_3 input; theta_ksi_est_err_tilt_1_3 output; ksi_est_err_squ_2_node_3 input; ksi_est_err_tilt_vec input; theta_ksi_est_err_tilt_2_3 output
function [theta_ksi_est_err_tilt_1_3, theta_ksi_est_err_tilt_2_3] = fcn(alfa_theta, ksi_est_err_squ_1_node_3, ksi_est_err_squ_2_node_3, ksi_est_err_tilt_vec)
%%%% 计算平滑递增函数
iiuav = 3;
theta_ksi_est_err_tilt_1_3 = ksi_est_err_squ_1_node_3(:) .* ( -1 + 2 ./ ( 1 + exp( -alfa_theta .* ksi_est_err_tilt_vec(:,iiuav) ) ) );
theta_ksi_est_err_tilt_2_3 = ksi_est_err_squ_2_node_3(:) .* ( -1 + 2 ./ ( 1 + exp( -alfa_theta .* ksi_est_err_tilt_vec(:,iiuav) ) ) );

== matlab function sim_tcyb_2024_pos_ctrl/cal theta_ksi_est_err_tilt agent 4 ==
  data: alfa_theta input; ksi_est_err_squ_1_node_4 input; theta_ksi_est_err_tilt_1_4 output; ksi_est_err_squ_2_node_4 input; ksi_est_err_tilt_vec input; theta_ksi_est_err_tilt_2_4 output
function [theta_ksi_est_err_tilt_1_4, theta_ksi_est_err_tilt_2_4] = fcn(alfa_theta, ksi_est_err_squ_1_node_4, ksi_est_err_squ_2_node_4, ksi_est_err_tilt_vec)
%%%% 计算平滑递增函数
iiuav = 4;
theta_ksi_est_err_tilt_1_4 = ksi_est_err_squ_1_node_4(:) .* ( -1 + 2 ./ ( 1 + exp( -alfa_theta .* ksi_est_err_tilt_vec(:,iiuav) ) ) );
theta_ksi_est_err_tilt_2_4 = ksi_est_err_squ_2_node_4(:) .* ( -1 + 2 ./ ( 1 + exp( -alfa_theta .* ksi_est_err_tilt_vec(:,iiuav) ) ) );

== matlab function sim_tcyb_2024_pos_ctrl/combine eps_p_hat adaptive ==
  data: eps_p_hat_1 input; eps_p_hat_vec output; eps_p_hat_2 input; eps_p_hat_3 input; eps_p_hat_4 input; eps_p_hat_5 input
function eps_p_hat_vec = fcn(eps_p_hat_1, eps_p_hat_2, eps_p_hat_3, eps_p_hat_4, eps_p_hat_5)
%%%% 合并领导者位置观测器输出结果
eps_p_hat_vec = [eps_p_hat_1, eps_p_hat_2, eps_p_hat_3, eps_p_hat_4, eps_p_hat_5];

== matlab function sim_tcyb_2024_pos_ctrl/cal theta_ksi_est_err_tilt agent 5 ==
  data: alfa_theta input; ksi_est_err_squ_1_node_5 input; theta_ksi_est_err_tilt_1_5 output; ksi_est_err_squ_2_node_5 input; ksi_est_err_tilt_vec input; theta_ksi_est_err_tilt_2_5 output
function [theta_ksi_est_err_tilt_1_5, theta_ksi_est_err_tilt_2_5] = fcn(alfa_theta, ksi_est_err_squ_1_node_5, ksi_est_err_squ_2_node_5, ksi_est_err_tilt_vec)
%%%% 计算平滑递增函数
iiuav = 5;
theta_ksi_est_err_tilt_1_5 = ksi_est_err_squ_1_node_5(:) .* ( -1 + 2 ./ ( 1 + exp( -alfa_theta .* ksi_est_err_tilt_vec(:,iiuav) ) ) );
theta_ksi_est_err_tilt_2_5 = ksi_est_err_squ_2_node_5(:) .* ( -1 + 2 ./ ( 1 + exp( -alfa_theta .* ksi_est_err_tilt_vec(:,iiuav) ) ) );

== matlab function sim_tcyb_2024_pos_ctrl/cal velocity estimate error ==
  data: eta_d_est_vec input; eta_est_err output; eta0 input; delta_eta_vec input
function eta_est_err  = fcn(eta_d_est_vec, eta0, delta_eta_vec)
%%%% 计算跟随者期望速度分布式观测器误差
eta_est_err = eta_d_est_vec - repmat(eta0, 1, 5) - delta_eta_vec;

== matlab function sim_tcyb_2024_pos_ctrl/choose eta_est_err_tilt 1 ==
  data: x input; y output
function y = fcn(x)
iiuav = 1;
y = x(:,iiuav);

== matlab function sim_tcyb_2024_pos_ctrl/choose eta_est_err_tilt 10 ==
  data: x input; y output
function y = fcn(x)
iiuav = 5;
y = x(:,iiuav);

== matlab function sim_tcyb_2024_pos_ctrl/choose eta_est_err_tilt 11 ==
  data: x input; y output
function y = fcn(x)
iiuav = 1;
y = x(:,iiuav);

== matlab function sim_tcyb_2024_pos_ctrl/choose eta_est_err_tilt 12 ==
  data: x input; y output
function y = fcn(x)
iiuav = 5;
y = x(:,iiuav);

== matlab function sim_tcyb_2024_pos_ctrl/choose eta_est_err_tilt 13 ==
  data: x input; y output
function y = fcn(x)
iiuav = 1;
y = x(:,iiuav);

== matlab function sim_tcyb_2024_pos_ctrl/choose eta_est_err_tilt 14 ==
  data: x input; y output
function y = fcn(x)
iiuav = 2;
y = x(:,iiuav);

== matlab function sim_tcyb_2024_pos_ctrl/choose eta_est_err_tilt 15 ==
  data: x input; y output
function y = fcn(x)
iiuav = 2;
y = x(:,iiuav);

== matlab function sim_tcyb_2024_pos_ctrl/choose eta_est_err_tilt 16 ==
  data: x input; y output
function y = fcn(x)
iiuav = 3;
y = x(:,iiuav);

== matlab function sim_tcyb_2024_pos_ctrl/choose eta_est_err_tilt 17 ==
  data: x input; y output
function y = fcn(x)
iiuav = 3;
y = x(:,iiuav);

== matlab function sim_tcyb_2024_pos_ctrl/choose eta_est_err_tilt 18 ==
  data: x input; y output
function y = fcn(x)
iiuav = 4;
y = x(:,iiuav);

== matlab function sim_tcyb_2024_pos_ctrl/choose eta_est_err_tilt 19 ==
  data: x input; y output
function y = fcn(x)
iiuav = 4;
y = x(:,iiuav);

== matlab function sim_tcyb_2024_pos_ctrl/choose eta_est_err_tilt 2 ==
  data: x input; y output
function y = fcn(x)
iiuav = 1;
y = x(:,iiuav);

== matlab function sim_tcyb_2024_pos_ctrl/choose eta_est_err_tilt 20 ==
  data: x input; y output
function y = fcn(x)
iiuav = 5;
y = x(:,iiuav);

== matlab function sim_tcyb_2024_pos_ctrl/eta_p_hat adaptive law agent 1 ==
  data: tau_p input; tsim input; d_eta_p_hat_1 output; err_lump_vec input; eta_p_hat_vec input
function d_eta_p_hat_1 = fcn(tau_p, tsim, err_lump_vec, eta_p_hat_vec)
%%%% 计算自适应律
iiuav = 1;
d_eta_p_hat_1 = tau_p * norm(err_lump_vec(:,iiuav), 2) ...
                                - ( 0.1 * exp(-tsim) ) * tau_p .* eta_p_hat_vec(iiuav);

== matlab function sim_tcyb_2024_pos_ctrl/choose eta_est_err_tilt 3 ==
  data: x input; y output
function y = fcn(x)
iiuav = 2;
y = x(:,iiuav);

== matlab function sim_tcyb_2024_pos_ctrl/choose eta_est_err_tilt 4 ==
  data: x input; y output
function y = fcn(x)
iiuav = 2;
y = x(:,iiuav);

== matlab function sim_tcyb_2024_pos_ctrl/choose eta_est_err_tilt 5 ==
  data: x input; y output
function y = fcn(x)
iiuav = 3;
y = x(:,iiuav);

== matlab function sim_tcyb_2024_pos_ctrl/choose eta_est_err_tilt 6 ==
  data: x input; y output
function y = fcn(x)
iiuav = 3;
y = x(:,iiuav);

== matlab function sim_tcyb_2024_pos_ctrl/choose eta_est_err_tilt 7 ==
  data: x input; y output
function y = fcn(x)
iiuav = 4;
y = x(:,iiuav);

== matlab function sim_tcyb_2024_pos_ctrl/choose eta_est_err_tilt 8 ==
  data: x input; y output
function y = fcn(x)
iiuav = 4;
y = x(:,iiuav);

== matlab function sim_tcyb_2024_pos_ctrl/choose eta_est_err_tilt 9 ==
  data: x input; y output
function y = fcn(x)
iiuav = 5;
y = x(:,iiuav);

== matlab function sim_tcyb_2024_pos_ctrl/combine follower desire velocity estimaters ==
  data: eta_d_est_1 input; eta_d_est_vec output; eta_d_est_2 input; eta_d_est_3 input; eta_d_est_4 input; eta_d_est_5 input
function eta_d_est_vec = fcn(eta_d_est_1, eta_d_est_2, eta_d_est_3, eta_d_est_4, eta_d_est_5)
%%%% 合并领导者位置观测器输出结果
eta_d_est_vec = [eta_d_est_1(:), eta_d_est_2(:), eta_d_est_3(:), eta_d_est_4(:), eta_d_est_5(:)];

== matlab function sim_tcyb_2024_pos_ctrl/combine leader position estimaters ==
  data: ksi_d_est_1 input; ksi_d_est_vec output; ksi_d_est_2 input; ksi_d_est_3 input; ksi_d_est_4 input; ksi_d_est_5 input
function ksi_d_est_vec  = fcn(ksi_d_est_1, ksi_d_est_2, ksi_d_est_3, ksi_d_est_4, ksi_d_est_5)
%%%% 合并领导者位置观测器输出结果
ksi_d_est_vec = [ksi_d_est_1(:), ksi_d_est_2(:), ksi_d_est_3(:), ksi_d_est_4(:), ksi_d_est_5(:)];

== matlab function sim_tcyb_2024_pos_ctrl/combine lumped follower observation error  ==
  data: ksi_est_err_tilt_1 input; ksi_est_err_tilt_2 input; ksi_est_err_tilt_3 input; ksi_est_err_tilt_4 input; ksi_est_err_tilt_5 input; ksi_est_err_tilt_vec output; eta_est_err_tilt_1 input; eta_est_err_tilt_vec output; eta_est_err_tilt_2 input; eta_est_err_tilt_3 input; eta_est_err_tilt_4 input; eta_est_err_tilt_5 input
function [ksi_est_err_tilt_vec, eta_est_err_tilt_vec]  = fcn(ksi_est_err_tilt_1, ksi_est_err_tilt_2, ksi_est_err_tilt_3, ksi_est_err_tilt_4, ksi_est_err_tilt_5, ...
                                                                                                        eta_est_err_tilt_1, eta_est_err_tilt_2, eta_est_err_tilt_3, eta_est_err_tilt_4, eta_est_err_tilt_5)
%%%% 合并领导者位置观测器输出结果
ksi_est_err_tilt_vec = [ksi_est_err_tilt_1, ksi_est_err_tilt_2, ksi_est_err_tilt_3, ksi_est_err_tilt_4, ksi_est_err_tilt_5];
eta_est_err_tilt_vec = [eta_est_err_tilt_1, eta_est_err_tilt_2, eta_est_err_tilt_3, eta_est_err_tilt_4, eta_est_err_tilt_5];

== matlab function sim_tcyb_2024_pos_ctrl/combine lumped follower position observation error ==
  data: theta_ksi_est_err_tilt_1_1 input; theta_ksi_est_err_tilt_1_2 input; theta_ksi_est_err_tilt_1_3 input; theta_ksi_est_err_tilt_1_4 input; theta_ksi_est_err_tilt_1_5 input; theta_ksi_est_err_tilt_1_vec output; theta_ksi_est_err_tilt_2_1 input; theta_ksi_est_err_tilt_2_vec output; theta_ksi_est_err_tilt_2_2 input; theta_ksi_est_err_tilt_2_3 input; theta_ksi_est_err_tilt_2_4 input; theta_ksi_est_err_tilt_2_5 input
function [theta_ksi_est_err_tilt_1_vec, theta_ksi_est_err_tilt_2_vec]  = fcn(theta_ksi_est_err_tilt_1_1, theta_ksi_est_err_tilt_1_2, theta_ksi_est_err_tilt_1_3, theta_ksi_est_err_tilt_1_4, theta_ksi_est_err_tilt_1_5, ...
                                                                                                                                    theta_ksi_est_err_tilt_2_1, theta_ksi_est_err_tilt_2_2, theta_ksi_est_err_tilt_2_3, theta_ksi_est_err_tilt_2_4, theta_ksi_est_err_tilt_2_5)
%%%% 合并领导者位置观测器输出结果
theta_ksi_est_err_tilt_1_vec = [theta_ksi_est_err_tilt_1_1(:), theta_ksi_est_err_tilt_1_2(:), theta_ksi_est_err_tilt_1_3(:), theta_ksi_est_err_tilt_1_4(:), theta_ksi_est_err_tilt_1_5(:)];
theta_ksi_est_err_tilt_2_vec = [theta_ksi_est_err_tilt_2_1(:), theta_ksi_est_err_tilt_2_2(:), theta_ksi_est_err_tilt_2_3(:), theta_ksi_est_err_tilt_2_4(:), theta_ksi_est_err_tilt_2_5(:)];

== matlab function sim_tcyb_2024_pos_ctrl/eta_p_hat adaptive law agent 2 ==
  data: tau_p input; tsim input; d_eta_p_hat_2 output; err_lump_vec input; eta_p_hat_vec input
function d_eta_p_hat_2 = fcn(tau_p, tsim, err_lump_vec, eta_p_hat_vec)
%%%% 计算自适应律
iiuav = 2;
d_eta_p_hat_2 = tau_p * norm(err_lump_vec(:,iiuav), 2) ...
                                - ( 0.1 * exp(-tsim) ) * tau_p .* eta_p_hat_vec(iiuav);

== matlab function sim_tcyb_2024_pos_ctrl/combine lumped follower velocity observation error ==
  data: theta_eta_est_err_tilt_1_1 input; theta_eta_est_err_tilt_1_2 input; theta_eta_est_err_tilt_1_3 input; theta_eta_est_err_tilt_1_4 input; theta_eta_est_err_tilt_1_5 input; theta_eta_est_err_tilt_1_vec output; theta_eta_est_err_tilt_2_1 input; theta_eta_est_err_tilt_2_vec output; theta_eta_est_err_tilt_2_2 input; theta_eta_est_err_tilt_2_3 input; theta_eta_est_err_tilt_2_4 input; theta_eta_est_err_tilt_2_5 input
function [theta_eta_est_err_tilt_1_vec, theta_eta_est_err_tilt_2_vec]  = fcn(theta_eta_est_err_tilt_1_1, theta_eta_est_err_tilt_1_2, theta_eta_est_err_tilt_1_3, theta_eta_est_err_tilt_1_4, theta_eta_est_err_tilt_1_5, ...
                                                                                                                                    theta_eta_est_err_tilt_2_1, theta_eta_est_err_tilt_2_2, theta_eta_est_err_tilt_2_3, theta_eta_est_err_tilt_2_4, theta_eta_est_err_tilt_2_5)
%%%% 合并领导者位置观测器输出结果
theta_eta_est_err_tilt_1_vec = [theta_eta_est_err_tilt_1_1(:), theta_eta_est_err_tilt_1_2(:), theta_eta_est_err_tilt_1_3(:), theta_eta_est_err_tilt_1_4(:), theta_eta_est_err_tilt_1_5(:)];
theta_eta_est_err_tilt_2_vec = [theta_eta_est_err_tilt_2_1(:), theta_eta_est_err_tilt_2_2(:), theta_eta_est_err_tilt_2_3(:), theta_eta_est_err_tilt_2_4(:), theta_eta_est_err_tilt_2_5(:)];

== matlab function sim_tcyb_2024_pos_ctrl/fixed-time distributed follower desire position observer agent 1 ==
  data: l1p input; d_ksi_d_est_1 output; l2p input; eta_d_est_vec input; theta_ksi_est_err_tilt_1_vec input; theta_ksi_est_err_tilt_2_vec input
function d_ksi_d_est_1 = fcn(l1p, l2p, eta_d_est_vec, theta_ksi_est_err_tilt_1_vec, theta_ksi_est_err_tilt_2_vec)
%%%% 固定时间跟随者期望位置分布式观测器
iiuav = 1;
d_ksi_d_est_1 = eta_d_est_vec(:,iiuav) - l1p * theta_ksi_est_err_tilt_1_vec(:,iiuav) - l2p * theta_ksi_est_err_tilt_2_vec(:,iiuav);

== matlab function sim_tcyb_2024_pos_ctrl/fixed-time distributed follower desire position observer agent 2 ==
  data: l1p input; d_ksi_d_est_2 output; l2p input; eta_d_est_vec input; theta_ksi_est_err_tilt_1_vec input; theta_ksi_est_err_tilt_2_vec input
function d_ksi_d_est_2 = fcn(l1p, l2p, eta_d_est_vec, theta_ksi_est_err_tilt_1_vec, theta_ksi_est_err_tilt_2_vec)
%%%% 固定时间跟随者期望位置分布式观测器
iiuav = 2;
d_ksi_d_est_2 = eta_d_est_vec(:,iiuav) - l1p * theta_ksi_est_err_tilt_1_vec(:,iiuav) - l2p * theta_ksi_est_err_tilt_2_vec(:,iiuav);

== matlab function sim_tcyb_2024_pos_ctrl/fixed-time distributed follower desire position observer agent 3 ==
  data: l1p input; d_ksi_d_est_3 output; l2p input; eta_d_est_vec input; theta_ksi_est_err_tilt_1_vec input; theta_ksi_est_err_tilt_2_vec input
function d_ksi_d_est_3 = fcn(l1p, l2p, eta_d_est_vec, theta_ksi_est_err_tilt_1_vec, theta_ksi_est_err_tilt_2_vec)
%%%% 固定时间跟随者期望位置分布式观测器
iiuav = 3;
d_ksi_d_est_3 = eta_d_est_vec(:,iiuav) - l1p * theta_ksi_est_err_tilt_1_vec(:,iiuav) - l2p * theta_ksi_est_err_tilt_2_vec(:,iiuav);

== matlab function sim_tcyb_2024_pos_ctrl/fixed-time distributed follower desire position observer agent 4 ==
  data: l1p input; d_ksi_d_est_4 output; l2p input; eta_d_est_vec input; theta_ksi_est_err_tilt_1_vec input; theta_ksi_est_err_tilt_2_vec input
function d_ksi_d_est_4 = fcn(l1p, l2p, eta_d_est_vec, theta_ksi_est_err_tilt_1_vec, theta_ksi_est_err_tilt_2_vec)
%%%% 固定时间跟随者期望位置分布式观测器
iiuav = 4;
d_ksi_d_est_4 = eta_d_est_vec(:,iiuav) - l1p * theta_ksi_est_err_tilt_1_vec(:,iiuav) - l2p * theta_ksi_est_err_tilt_2_vec(:,iiuav);

== matlab function sim_tcyb_2024_pos_ctrl/fixed-time distributed follower desire position observer agent 5 ==
  data: l1p input; d_ksi_d_est_5 output; l2p input; eta_d_est_vec input; theta_ksi_est_err_tilt_1_vec input; theta_ksi_est_err_tilt_2_vec input
function d_ksi_d_est_5 = fcn(l1p, l2p, eta_d_est_vec, theta_ksi_est_err_tilt_1_vec, theta_ksi_est_err_tilt_2_vec)
%%%% 固定时间跟随者期望位置分布式观测器
iiuav = 5;
d_ksi_d_est_5 = eta_d_est_vec(:,iiuav) - l1p * theta_ksi_est_err_tilt_1_vec(:,iiuav) - l2p * theta_ksi_est_err_tilt_2_vec(:,iiuav);

== matlab function sim_tcyb_2024_pos_ctrl/fixed-time distributed follower desire velocity observer agent 1 ==
  data: l1v input; d_eta_d_est_1 output; l2v input; theta_eta_est_err_tilt_1_vec input; theta_eta_est_err_tilt_2_vec input
function d_eta_d_est_1 = fcn(l1v, l2v, theta_eta_est_err_tilt_1_vec, theta_eta_est_err_tilt_2_vec)
%%%% 固定时间跟随者期望速度分布式观测器
iiuav = 1;
d_eta_d_est_1 = -l1v * theta_eta_est_err_tilt_1_vec(:,iiuav) - l2v * theta_eta_est_err_tilt_2_vec(:,iiuav);

== matlab function sim_tcyb_2024_pos_ctrl/fixed-time distributed follower desire velocity observer agent 2 ==
  data: l1v input; d_eta_d_est_2 output; l2v input; theta_eta_est_err_tilt_1_vec input; theta_eta_est_err_tilt_2_vec input
function d_eta_d_est_2 = fcn(l1v, l2v, theta_eta_est_err_tilt_1_vec, theta_eta_est_err_tilt_2_vec)
%%%% 固定时间跟随者期望速度分布式观测器
iiuav = 2;
d_eta_d_est_2 = -l1v * theta_eta_est_err_tilt_1_vec(:,iiuav) - l2v * theta_eta_est_err_tilt_2_vec(:,iiuav);

== matlab function sim_tcyb_2024_pos_ctrl/fixed-time distributed follower desire velocity observer agent 3 ==
  data: l1v input; d_eta_d_est_3 output; l2v input; theta_eta_est_err_tilt_1_vec input; theta_eta_est_err_tilt_2_vec input
function d_eta_d_est_3 = fcn(l1v, l2v, theta_eta_est_err_tilt_1_vec, theta_eta_est_err_tilt_2_vec)
%%%% 固定时间跟随者期望速度分布式观测器
iiuav = 3;
d_eta_d_est_3 = -l1v * theta_eta_est_err_tilt_1_vec(:,iiuav) - l2v * theta_eta_est_err_tilt_2_vec(:,iiuav);

== matlab function sim_tcyb_2024_pos_ctrl/eta_p_hat adaptive law agent 3 ==
  data: tau_p input; tsim input; d_eta_p_hat_3 output; err_lump_vec input; eta_p_hat_vec input
function d_eta_p_hat_3 = fcn(tau_p, tsim, err_lump_vec, eta_p_hat_vec)
%%%% 计算自适应律
iiuav = 3;
d_eta_p_hat_3 = tau_p * norm(err_lump_vec(:,iiuav), 2) ...
                                - ( 0.1 * exp(-tsim) ) * tau_p .* eta_p_hat_vec(iiuav);

== matlab function sim_tcyb_2024_pos_ctrl/fixed-time distributed follower desire velocity observer agent 4 ==
  data: l1v input; d_eta_d_est_4 output; l2v input; theta_eta_est_err_tilt_1_vec input; theta_eta_est_err_tilt_2_vec input
function d_eta_d_est_4 = fcn(l1v, l2v, theta_eta_est_err_tilt_1_vec, theta_eta_est_err_tilt_2_vec)
%%%% 固定时间跟随者期望速度分布式观测器
iiuav = 4;
d_eta_d_est_4 = -l1v * theta_eta_est_err_tilt_1_vec(:,iiuav) - l2v * theta_eta_est_err_tilt_2_vec(:,iiuav);

== matlab function sim_tcyb_2024_pos_ctrl/fixed-time distributed follower desire velocity observer agent 5 ==
  data: l1v input; d_eta_d_est_5 output; l2v input; theta_eta_est_err_tilt_1_vec input; theta_eta_est_err_tilt_2_vec input
function d_eta_d_est_5 = fcn(l1v, l2v, theta_eta_est_err_tilt_1_vec, theta_eta_est_err_tilt_2_vec)
%%%% 固定时间跟随者期望速度分布式观测器
iiuav = 5;
d_eta_d_est_5 = -l1v * theta_eta_est_err_tilt_1_vec(:,iiuav) - l2v * theta_eta_est_err_tilt_2_vec(:,iiuav);

== matlab function sim_tcyb_2024_pos_ctrl/trans to column41 ==
  data: x input; y output
function y = fcn(x)
y = x(:);

== matlab function sim_tcyb_2024_pos_ctrl/trans to column42 ==
  data: x input; y output
function y = fcn(x)
y = x(:);

== matlab function sim_tcyb_2024_pos_ctrl/trans to column43 ==
  data: x input; y output
function y = fcn(x)
y = x(:);

== matlab function sim_tcyb_2024_pos_ctrl/trans to column44 ==
  data: x input; y output
function y = fcn(x)
y = x(:);

== matlab function sim_tcyb_2024_pos_ctrl/trans to column45 ==
  data: x input; y output
function y = fcn(x)
y = x(:);

== matlab function sim_tcyb_2024_pos_ctrl/trans to column46 ==
  data: x input; y output
function y = fcn(x)
y = x(:);

== matlab function sim_tcyb_2024_pos_ctrl/trans to column47 ==
  data: x input; y output
function y = fcn(x)
y = x(:);

== matlab function sim_tcyb_2024_pos_ctrl/trans to column48 ==
  data: x input; y output
function y = fcn(x)
y = x(:);

== matlab function sim_tcyb_2024_pos_ctrl/trans to column49 ==
  data: x input; y output
function y = fcn(x)
y = x(:);

== matlab function sim_tcyb_2024_pos_ctrl/trans to column50 ==
  data: x input; y output
function y = fcn(x)
y = x(:);
